simulink model "spherical_wrist"  (R2024b)
settings: Solver=ode23t  StartTime=0.0  StopTime=100  FixedStep=0.001  RelTol=1e-3
InitFcn:
  | % WRIST_mk2_1_DataFile
  | IC_021_G_207_MECH_DataFile
model workspace (MAT data in the model file):
  Damp : Simulink.Parameter (value not decoded)
  Dm : Simulink.Parameter (value not decoded)
  Jm : Simulink.Parameter (value not decoded)
  Km : Simulink.Parameter (value not decoded)
  Tc : Simulink.Parameter (value not decoded)
symbols that are objects in the model workspace (value not decoded): Damp, Dm, Tc
undefined symbols (not defined in the file or in its folder): smiData, X, Y, Z
libraries: sm_lib x370, nesl_utility x32, fl_lib x15, sdl_lib x9, simulink_extras x4, simulink x3, sharedtransform x2, slpidlib x1
(part 10 of 10)

== system spherical_wrist/NewWrist21/ROD 3/SPINA ROD 3 ==
  ReferenceFrame : sm_lib/Frames and Transforms/Reference Frame
  Solid : sm_lib/Body Elements/File Solid  ExtGeomFileName=ic_021_p_196_prt.step  UnitType=FromFile  ExtGeomFileUnits=m  StepReaderType=HEX  ExportConvexHullGeometry=off  InertiaType=Custom  BasedOnType=DensityFromFile  Density=1000  DensityUnits=kg/m^3  Mass=smiData.Solid(5).mass  MassUnits=kg  CenterOfMass=smiData.Solid(5).CoM  CenterOfMassUnits=mm  MomentsOfInertia=smiData.Solid(5).MoI  MomentsOfInertiaUnits=kg*mm^2  ProductsOfInertia=smiData.Solid(5).PoI  ProductsOfInertiaUnits=kg*mm^2  GraphicType=FromGeometry  MarkerShape=Sphere  MarkerSize=10  GraphicVisPropType=SimpleVisualProperties  GraphicDiffuseColor=smiData.Solid(5).color  GraphicOpacity=smiData.Solid(5).opacity  GraphicSpecularColor=[0.5 0.5 0.5 1.0]  GraphicAmbientColor=[0.15 0.15 0.15 1.0]  GraphicEmissiveColor=[0.0 0.0 0.0 1.0]  GraphicShininess=75  DoExposeReferenceFrame=on  SerializedFrames=<Frames/>
  Transform : sm_lib/Frames and Transforms/Rigid Transform  RotationMethod=ArbitraryAxis  FollAlignAxisA=+X  BaseAlignAxisA=+Y  FollAlignAxisB=+Y  BaseAlignAxisB=+Z  RotationStandardAxis=+Z  RotationAngle=smiData.RigidTransform(8).angle  RotationAngleUnits=rad  RotationArbitraryAxis=smiData.RigidTransform(8).axis  RotationSequenceAxes=FollowerAxes  RotationSequence=XYX  RotationSequenceAngles=[0 0 0]  RotationSequenceAnglesUnits=deg  RotationMatrix=[1 0 0;0 1 0;0 0 1]  Quaternion=[1 0 0 0]  TranslationMethod=Cartesian  TranslationCartesianOffset=smiData.RigidTransform(8).translation  TranslationCartesianOffsetUnits=mm  TranslationStandardAxis=+Z  TranslationStandardOffset=0  TranslationStandardOffsetUnits=m  TranslationROffset=0  TranslationROffsetUnits=m  TranslationThetaOffset=0  TranslationThetaOffsetUnits=deg  TranslationZOffset=0  TranslationZOffsetUnits=m
  F : PMIOPort  Side=Left
  connections:
  Solid/RConn1 -- ReferenceFrame/RConn1 -- Transform/LConn1
  Transform/RConn1 -- F/RConn1

== system spherical_wrist/NewWrist21/ROD 3/x618_4_RIGID ==
  ReferenceFrame : sm_lib/Frames and Transforms/Reference Frame
  Solid : sm_lib/Body Elements/File Solid  ExtGeomFileName=618-4_prt.step  UnitType=FromFile  ExtGeomFileUnits=m  StepReaderType=HEX  ExportConvexHullGeometry=off  InertiaType=Custom  BasedOnType=DensityFromFile  Density=1000  DensityUnits=kg/m^3  Mass=smiData.Solid(4).mass  MassUnits=kg  CenterOfMass=smiData.Solid(4).CoM  CenterOfMassUnits=mm  MomentsOfInertia=smiData.Solid(4).MoI  MomentsOfInertiaUnits=kg*mm^2  ProductsOfInertia=smiData.Solid(4).PoI  ProductsOfInertiaUnits=kg*mm^2  GraphicType=FromGeometry  MarkerShape=Sphere  MarkerSize=10  GraphicVisPropType=SimpleVisualProperties  GraphicDiffuseColor=smiData.Solid(4).color  GraphicOpacity=smiData.Solid(4).opacity  GraphicSpecularColor=[0.5 0.5 0.5 1.0]  GraphicAmbientColor=[0.15 0.15 0.15 1.0]  GraphicEmissiveColor=[0.0 0.0 0.0 1.0]  GraphicShininess=75  DoExposeReferenceFrame=on  SerializedFrames=<Frames/>
  F : PMIOPort  Side=Left
  connections:
  Solid/RConn1 -- ReferenceFrame/RConn1 -- F/RConn1

== system spherical_wrist/NewWrist21/ROD 3/x618_4_RIGID1 ==
  ReferenceFrame : sm_lib/Frames and Transforms/Reference Frame
  Solid : sm_lib/Body Elements/File Solid  ExtGeomFileName=618-4_prt.step  UnitType=FromFile  ExtGeomFileUnits=m  StepReaderType=HEX  ExportConvexHullGeometry=off  InertiaType=Custom  BasedOnType=DensityFromFile  Density=1000  DensityUnits=kg/m^3  Mass=smiData.Solid(4).mass  MassUnits=kg  CenterOfMass=smiData.Solid(4).CoM  CenterOfMassUnits=mm  MomentsOfInertia=smiData.Solid(4).MoI  MomentsOfInertiaUnits=kg*mm^2  ProductsOfInertia=smiData.Solid(4).PoI  ProductsOfInertiaUnits=kg*mm^2  GraphicType=FromGeometry  MarkerShape=Sphere  MarkerSize=10  GraphicVisPropType=SimpleVisualProperties  GraphicDiffuseColor=smiData.Solid(4).color  GraphicOpacity=smiData.Solid(4).opacity  GraphicSpecularColor=[0.5 0.5 0.5 1.0]  GraphicAmbientColor=[0.15 0.15 0.15 1.0]  GraphicEmissiveColor=[0.0 0.0 0.0 1.0]  GraphicShininess=75  DoExposeReferenceFrame=on  SerializedFrames=<Frames/>
  F : PMIOPort  Side=Left
  connections:
  Solid/RConn1 -- ReferenceFrame/RConn1 -- F/RConn1

== system spherical_wrist/NewWrist21/ROD 3/x618_4_RIGID2 ==
  ReferenceFrame : sm_lib/Frames and Transforms/Reference Frame
  Solid : sm_lib/Body Elements/File Solid  ExtGeomFileName=618-4_prt.step  UnitType=FromFile  ExtGeomFileUnits=m  StepReaderType=HEX  ExportConvexHullGeometry=off  InertiaType=Custom  BasedOnType=DensityFromFile  Density=1000  DensityUnits=kg/m^3  Mass=smiData.Solid(4).mass  MassUnits=kg  CenterOfMass=smiData.Solid(4).CoM  CenterOfMassUnits=mm  MomentsOfInertia=smiData.Solid(4).MoI  MomentsOfInertiaUnits=kg*mm^2  ProductsOfInertia=smiData.Solid(4).PoI  ProductsOfInertiaUnits=kg*mm^2  GraphicType=FromGeometry  MarkerShape=Sphere  MarkerSize=10  GraphicVisPropType=SimpleVisualProperties  GraphicDiffuseColor=smiData.Solid(4).color  GraphicOpacity=smiData.Solid(4).opacity  GraphicSpecularColor=[0.5 0.5 0.5 1.0]  GraphicAmbientColor=[0.15 0.15 0.15 1.0]  GraphicEmissiveColor=[0.0 0.0 0.0 1.0]  GraphicShininess=75  DoExposeReferenceFrame=on  SerializedFrames=<Frames/>
  Transform : sm_lib/Frames and Transforms/Rigid Transform  RotationMethod=ArbitraryAxis  FollAlignAxisA=+X  BaseAlignAxisA=+Y  FollAlignAxisB=+Y  BaseAlignAxisB=+Z  RotationStandardAxis=+Z  RotationAngle=smiData.RigidTransform(34).angle  RotationAngleUnits=rad  RotationArbitraryAxis=smiData.RigidTransform(34).axis  RotationSequenceAxes=FollowerAxes  RotationSequence=XYX  RotationSequenceAngles=[0 0 0]  RotationSequenceAnglesUnits=deg  RotationMatrix=[1 0 0;0 1 0;0 0 1]  Quaternion=[1 0 0 0]  TranslationMethod=Cartesian  TranslationCartesianOffset=smiData.RigidTransform(34).translation  TranslationCartesianOffsetUnits=mm  TranslationStandardAxis=+Z  TranslationStandardOffset=0  TranslationStandardOffsetUnits=m  TranslationROffset=0  TranslationROffsetUnits=m  TranslationThetaOffset=0  TranslationThetaOffsetUnits=deg  TranslationZOffset=0  TranslationZOffsetUnits=m
  Transform1 : sm_lib/Frames and Transforms/Rigid Transform  RotationMethod=ArbitraryAxis  FollAlignAxisA=+X  BaseAlignAxisA=+Y  FollAlignAxisB=+Y  BaseAlignAxisB=+Z  RotationStandardAxis=+Z  RotationAngle=smiData.RigidTransform(51).angle  RotationAngleUnits=rad  RotationArbitraryAxis=smiData.RigidTransform(51).axis  RotationSequenceAxes=FollowerAxes  RotationSequence=XYX  RotationSequenceAngles=[0 0 0]  RotationSequenceAnglesUnits=deg  RotationMatrix=[1 0 0;0 1 0;0 0 1]  Quaternion=[1 0 0 0]  TranslationMethod=Cartesian  TranslationCartesianOffset=smiData.RigidTransform(51).translation  TranslationCartesianOffsetUnits=mm  TranslationStandardAxis=+Z  TranslationStandardOffset=0  TranslationStandardOffsetUnits=m  TranslationROffset=0  TranslationROffsetUnits=m  TranslationThetaOffset=0  TranslationThetaOffsetUnits=deg  TranslationZOffset=0  TranslationZOffsetUnits=m
  F1 : PMIOPort  Side=Left
  F : PMIOPort  Port=2  Side=Left
  connections:
  Solid/RConn1 -- ReferenceFrame/RConn1 -- Transform/LConn1 -- Transform1/LConn1
  Transform/RConn1 -- F/RConn1
  Transform1/RConn1 -- F1/RConn1

== system spherical_wrist/NewWrist21/ROD 3/x618_4_RIGID3 ==
  ReferenceFrame : sm_lib/Frames and Transforms/Reference Frame
  Solid : sm_lib/Body Elements/File Solid  ExtGeomFileName=618-4_prt.step  UnitType=FromFile  ExtGeomFileUnits=m  StepReaderType=HEX  ExportConvexHullGeometry=off  InertiaType=Custom  BasedOnType=DensityFromFile  Density=1000  DensityUnits=kg/m^3  Mass=smiData.Solid(4).mass  MassUnits=kg  CenterOfMass=smiData.Solid(4).CoM  CenterOfMassUnits=mm  MomentsOfInertia=smiData.Solid(4).MoI  MomentsOfInertiaUnits=kg*mm^2  ProductsOfInertia=smiData.Solid(4).PoI  ProductsOfInertiaUnits=kg*mm^2  GraphicType=FromGeometry  MarkerShape=Sphere  MarkerSize=10  GraphicVisPropType=SimpleVisualProperties  GraphicDiffuseColor=smiData.Solid(4).color  GraphicOpacity=smiData.Solid(4).opacity  GraphicSpecularColor=[0.5 0.5 0.5 1.0]  GraphicAmbientColor=[0.15 0.15 0.15 1.0]  GraphicEmissiveColor=[0.0 0.0 0.0 1.0]  GraphicShininess=75  DoExposeReferenceFrame=on  SerializedFrames=<Frames/>
  Transform : sm_lib/Frames and Transforms/Rigid Transform  RotationMethod=ArbitraryAxis  FollAlignAxisA=+X  BaseAlignAxisA=+Y  FollAlignAxisB=+Y  BaseAlignAxisB=+Z  RotationStandardAxis=+Z  RotationAngle=smiData.RigidTransform(46).angle  RotationAngleUnits=rad  RotationArbitraryAxis=smiData.RigidTransform(46).axis  RotationSequenceAxes=FollowerAxes  RotationSequence=XYX  RotationSequenceAngles=[0 0 0]  RotationSequenceAnglesUnits=deg  RotationMatrix=[1 0 0;0 1 0;0 0 1]  Quaternion=[1 0 0 0]  TranslationMethod=Cartesian  TranslationCartesianOffset=smiData.RigidTransform(46).translation  TranslationCartesianOffsetUnits=mm  TranslationStandardAxis=+Z  TranslationStandardOffset=0  TranslationStandardOffsetUnits=m  TranslationROffset=0  TranslationROffsetUnits=m  TranslationThetaOffset=0  TranslationThetaOffsetUnits=deg  TranslationZOffset=0  TranslationZOffsetUnits=m
  Transform1 : sm_lib/Frames and Transforms/Rigid Transform  RotationMethod=ArbitraryAxis  FollAlignAxisA=+X  BaseAlignAxisA=+Y  FollAlignAxisB=+Y  BaseAlignAxisB=+Z  RotationStandardAxis=+Z  RotationAngle=smiData.RigidTransform(57).angle  RotationAngleUnits=rad  RotationArbitraryAxis=smiData.RigidTransform(57).axis  RotationSequenceAxes=FollowerAxes  RotationSequence=XYX  RotationSequenceAngles=[0 0 0]  RotationSequenceAnglesUnits=deg  RotationMatrix=[1 0 0;0 1 0;0 0 1]  Quaternion=[1 0 0 0]  TranslationMethod=Cartesian  TranslationCartesianOffset=smiData.RigidTransform(57).translation  TranslationCartesianOffsetUnits=mm  TranslationStandardAxis=+Z  TranslationStandardOffset=0  TranslationStandardOffsetUnits=m  TranslationROffset=0  TranslationROffsetUnits=m  TranslationThetaOffset=0  TranslationThetaOffsetUnits=deg  TranslationZOffset=0  TranslationZOffsetUnits=m
  F1 : PMIOPort  Side=Left
  F : PMIOPort  Port=2  Side=Left
  connections:
  Solid/RConn1 -- ReferenceFrame/RConn1 -- Transform/LConn1 -- Transform1/LConn1
  Transform/RConn1 -- F/RConn1
  Transform1/RConn1 -- F1/RConn1

== system spherical_wrist/Position_Controller/wrapTo180Simulink/singleWrapTo180_1 ==
  angle : Inport
  Add6 : Sum  Inputs=-+
  Add7 : Sum
  Constant : Constant  Value=360
  Constant4 : Constant  Value=180
  Constant5 : Constant  Value=360
  Constant6 : Constant  Value=-180
  Relational Operator : RelationalOperator  Operator=>  OutDataTypeStr=boolean  RndMeth=Simplest  InputSameDT=off
  Relational Operator1 : RelationalOperator  Operator=<  OutDataTypeStr=boolean  RndMeth=Simplest  InputSameDT=off
  Switch4 : Switch  Criteria=u2 > Threshold  SaturateOnIntegerOverflow=off  InputSameDT=off
  Switch5 : Switch  Criteria=u2 > Threshold  SaturateOnIntegerOverflow=off  InputSameDT=off
  wrappedAngle : Outport
  wires:
  Relational Operator/1 -> Switch4/2
  Constant5/1 -> Add6/1
  Switch5/1 -> wrappedAngle/1
  Add7/1 -> Switch5/1
  Constant4/1 -> Relational Operator/2
  Switch4/1 -> Switch5/3
  Constant/1 -> Add7/2
  Add6/1 -> Switch4/1
  angle/1 -> Switch4/3, Relational Operator/1, Add6/2, Add7/1, Relational Operator1/1
  Constant6/1 -> Relational Operator1/2
  Relational Operator1/1 -> Switch5/2

== system spherical_wrist/Position_Controller/wrapTo180Simulink/singleWrapTo180_2 ==
  angle : Inport
  Add6 : Sum  Inputs=-+
  Add7 : Sum
  Constant : Constant  Value=360
  Constant4 : Constant  Value=180
  Constant5 : Constant  Value=360
  Constant6 : Constant  Value=-180
  Relational Operator : RelationalOperator  Operator=>  OutDataTypeStr=boolean  RndMeth=Simplest  InputSameDT=off
  Relational Operator1 : RelationalOperator  Operator=<  OutDataTypeStr=boolean  RndMeth=Simplest  InputSameDT=off
  Switch4 : Switch  Criteria=u2 > Threshold  SaturateOnIntegerOverflow=off  InputSameDT=off
  Switch5 : Switch  Criteria=u2 > Threshold  SaturateOnIntegerOverflow=off  InputSameDT=off
  wrappedAngle : Outport
  wires:
  Relational Operator/1 -> Switch4/2
  Constant5/1 -> Add6/1
  Switch5/1 -> wrappedAngle/1
  Add7/1 -> Switch5/1
  Constant4/1 -> Relational Operator/2
  Switch4/1 -> Switch5/3
  Constant/1 -> Add7/2
  Add6/1 -> Switch4/1
  angle/1 -> Switch4/3, Relational Operator/1, Add6/2, Add7/1, Relational Operator1/1
  Constant6/1 -> Relational Operator1/2
  Relational Operator1/1 -> Switch5/2

== system spherical_wrist/Position_Controller/wrapTo180Simulink/singleWrapTo180_3 ==
  angle : Inport
  Add6 : Sum  Inputs=-+
  Add7 : Sum
  Constant : Constant  Value=360
  Constant4 : Constant  Value=180
  Constant5 : Constant  Value=360
  Constant6 : Constant  Value=-180
  Relational Operator : RelationalOperator  Operator=>  OutDataTypeStr=boolean  RndMeth=Simplest  InputSameDT=off
  Relational Operator1 : RelationalOperator  Operator=<  OutDataTypeStr=boolean  RndMeth=Simplest  InputSameDT=off
  Switch4 : Switch  Criteria=u2 > Threshold  SaturateOnIntegerOverflow=off  InputSameDT=off
  Switch5 : Switch  Criteria=u2 > Threshold  SaturateOnIntegerOverflow=off  InputSameDT=off
  wrappedAngle : Outport
  wires:
  Relational Operator/1 -> Switch4/2
  Constant5/1 -> Add6/1
  Switch5/1 -> wrappedAngle/1
  Add7/1 -> Switch5/1
  Constant4/1 -> Relational Operator/2
  Switch4/1 -> Switch5/3
  Constant/1 -> Add7/2
  Add6/1 -> Switch4/1
  angle/1 -> Switch4/3, Relational Operator/1, Add6/2, Add7/1, Relational Operator1/1
  Constant6/1 -> Relational Operator1/2
  Relational Operator1/1 -> Switch5/2

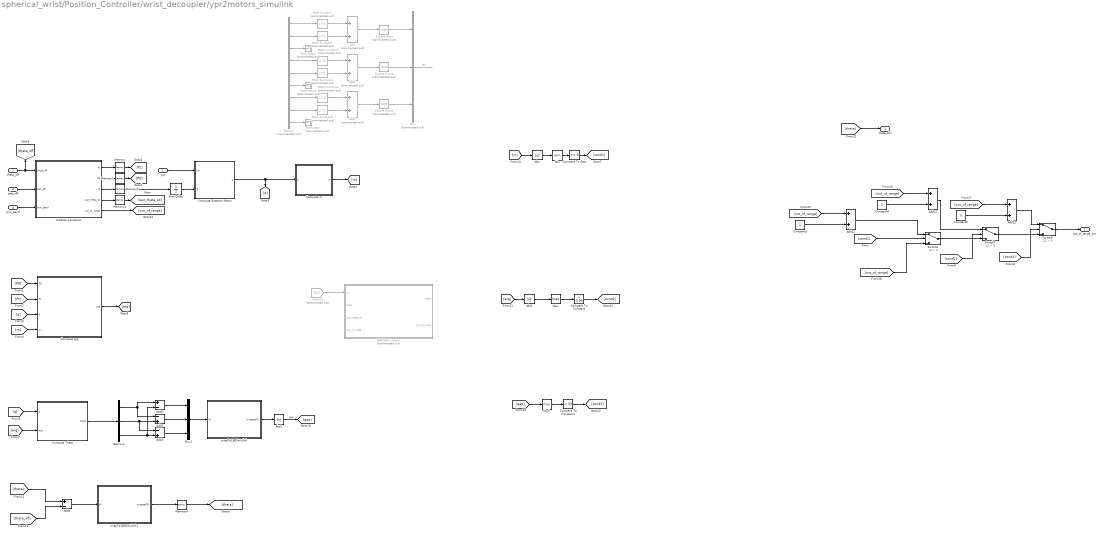
== system spherical_wrist/Position_Controller/wrist_decoupler/ypr2motors_simulink ==
  ypr : Inport
  theta_off : Inport  Port=2
  plat_off : Inport  Port=3
  arm_bend : Inport  Port=4
  Abs : Abs  SaturateOnIntegerOverflow=off
  Abs1 : Abs  SaturateOnIntegerOverflow=off
  Abs2 : Abs  SaturateOnIntegerOverflow=off
  Add : Sum  Commented=on
  Add1 : Sum  Commented=on
  Add11 : Sum
  Add12 : Sum
  Add13 : Sum
  Add2 : Sum  Commented=on
  Add3 : Sum  Inputs=-+
  Add4 : Sum  Inputs=-+
  Add5 : Sum  Inputs=+-
  Add6 : Sum  Inputs=+-
  Compare To Constant : simulink/Logic and Bit Operations/Compare To Constant  relop=>  const=0.99  OutDataTypeStr=boolean
  Compare To Constant1 : simulink/Logic and Bit Operations/Compare To Constant  relop=<  const=33  OutDataTypeStr=boolean
  Compare To Zero : simulink/Logic and Bit Operations/Compare To Zero  relop===  OutDataTypeStr=boolean
  Compute Rotation Matrix : MATLAB Function  TreatAsAtomicUnit=on
      settings: MinAlgLoopOccurrences=on
  Compute Theta : MATLAB Function  TreatAsAtomicUnit=on
  Compute arg : MATLAB Function  TreatAsAtomicUnit=on
      settings: MinAlgLoopOccurrences=on
  Compute m : MATLAB Function  TreatAsAtomicUnit=on
  Constant3 : Constant
  Constant4 : Constant  Value=2
  Constant5 : Constant  Value=3
  Demux : Demux  Commented=on  Outputs=9
  Demux1 : Demux  Outputs=3
  From24 : From  Commented=on  GotoTag=m
  Initialize Constants : MATLAB Function  TreatAsAtomicUnit=on
      settings: MinAlgLoopOccurrences=on
  MATLAB Function : MATLAB Function  Commented=on  TreatAsAtomicUnit=on
  Math Function{,1..5} (6 alike) : Math  Commented=on  Operator=square
  Max : MinMax  Function=max
  Memory{,1..4} (5 alike) : Memory  InheritSampleTime=on
  Min : MinMax
  Min1 : MinMax
  Mux : Mux  Commented=on  Inputs=3
  Mux1 : Mux  Inputs=3
  Square Root : Sqrt  Commented=on
  Square Root1 : Sqrt  Commented=on
  Square Root2 : Sqrt  Commented=on
  Switch6 : Switch  Criteria=u2 > Threshold  SaturateOnIntegerOverflow=off  InputSameDT=off
  Switch7 : Switch  Criteria=u2 > Threshold  SaturateOnIntegerOverflow=off  InputSameDT=off
  Switch8 : Switch  Criteria=u2 > Threshold  SaturateOnIntegerOverflow=off  InputSameDT=off
  Terminator : Terminator  Commented=on
  Terminator1 : Terminator  Commented=on
  Terminator2 : Terminator  Commented=on
  Unit Delay : UnitDelay  SampleTime=-1  HasFrameUpgradeWarning=on
  wrapTo180Simulink : Subsystem
  wrapTo180Simulink1 : Subsystem
  theta_sim : Outport
  out_of_range_sim : Outport  Port=2
  wires:
  theta_off/1 -> Initialize Constants/1(theta_off), [theta_off]
  plat_off/1 -> Initialize Constants/2(plat_off)
  arm_bend/1 -> Initialize Constants/3(arm_bend)
  Initialize Constants/1(Pz) -> Memory/1
  Initialize Constants/2(PQ) -> Memory1/1
  Initialize Constants/3(Q) -> Memory2/1
  ypr/1 -> Compute Rotation Matrix/1(ypr)
  Memory2/1 -> Unit Delay/1
  Memory1/1 -> [PQ]
  Memory/1 -> [Pz]
  [Pz] -> Compute arg/2(Pz)
  Compute Rotation Matrix/1(q) -> Compute m/1(q), [q]
  [q] -> Compute arg/3(q)
  [m] -> Compute arg/4(m)
  Compute arg/1(arg) -> [arg]
  [q] -> Compute Theta/1(q)
  [arg] -> Compute Theta/2(arg)
  Compute Theta/1(theta) -> Demux1/1
  Demux1/2 -> Add4/1, Add3/2
  Demux1/1 -> Add3/1, Add5/1
  Demux1/3 -> Add5/2, Add4/2
  Add5/1 -> Mux1/1
  Add3/1 -> Mux1/2
  Add4/1 -> Mux1/3
  Mux1/1 -> wrapTo180Simulink/1(th)
  [theta] -> Add6/1
  [theta_off] -> Add6/2
  Add6/1 -> wrapTo180Simulink1/1(th)
  wrapTo180Simulink1/1(wrappedTh) -> Memory4/1
  Memory4/1 -> [theta]
  Initialize Constants/4(last_theta_ok) -> Memory3/1
  Memory3/1 -> [last_theta_ok]
  [theta] -> theta_sim/1
  Initialize Constants/5(out_of_range) -> [out_of_range]
  Min/1 -> Compare To Zero/1
  Compare To Zero/1 -> [cond1]
  Abs/1 -> Min/1
  [m] -> Abs/1
  Abs1/1 -> Max/1
  Max/1 -> Compare To Constant/1
  Compare To Constant/1 -> [cond2]
  [arg] -> Abs1/1
  Min1/1 -> Compare To Constant1/1
  Compare To Constant1/1 -> [cond3]
  wrapTo180Simulink/1(wrappedTh) -> Abs2/1
  Abs2/1 -> [gap]  "gap"
  [gap] -> Min1/1
  From24/1 -> MATLAB Function/1(m)
  Constant3/1 -> Add11/2
  [out_of_range] -> Add11/1
  Add11/1 -> Switch6/1
  Switch6/1 -> Switch7/3
  Switch7/1 -> Switch8/3
  [out_of_range] -> Add12/1
  Add12/1 -> Switch7/1
  Constant4/1 -> Add12/2
  [out_of_range] -> Add13/1
  Add13/1 -> Switch8/1
  Constant5/1 -> Add13/2
  Switch8/1 -> out_of_range_sim/1
  [out_of_range] -> Switch6/3
  [cond1] -> Switch6/2
  [cond2] -> Switch7/2
  [cond3] -> Switch8/2
  Add/1 -> Square Root/1
  Square Root1/1 -> Mux/2
  Demux/3 -> Terminator2/1
  Demux/9 -> Terminator/1
  Square Root/1 -> Mux/1
  Square Root2/1 -> Mux/3
  Math Function/1 -> Add/1
  Math Function1/1 -> Add/2
  Demux/6 -> Terminator1/1
  Math Function2/1 -> Add1/1
  Mux/1 -> ?  "m"
  Demux/7 -> Math Function4/1
  Demux/4 -> Math Function2/1
  Demux/8 -> Math Function5/1
  Demux/1 -> Math Function/1
  Demux/5 -> Math Function3/1
  Math Function4/1 -> Add2/1
  Math Function3/1 -> Add1/2
  ? -> Demux/1
  Add1/1 -> Square Root1/1
  Add2/1 -> Square Root2/1
  Demux/2 -> Math Function1/1
  Math Function5/1 -> Add2/2
  Compute m/1(m) -> [m]
  Unit Delay/1 -> Compute Rotation Matrix/2(Q)
  [PQ] -> Compute arg/1(PQ)

== system spherical_wrist/Position_Controller/wrist_decoupler/ypr2motors_simulink/wrapTo180Simulink ==
  th : Inport
  Demux : Demux  Outputs=3
  Mux : Mux  Inputs=3
  singleWrapTo180_1 : Subsystem
  singleWrapTo180_2 : Subsystem
  singleWrapTo180_3 : Subsystem
  wrappedTh : Outport
  wires:
  singleWrapTo180_1/1(wrappedAngle) -> Mux/1
  singleWrapTo180_3/1(wrappedAngle) -> Mux/3
  singleWrapTo180_2/1(wrappedAngle) -> Mux/2
  Demux/3 -> singleWrapTo180_3/1(angle)
  th/1 -> Demux/1
  Demux/1 -> singleWrapTo180_1/1(angle)
  Demux/2 -> singleWrapTo180_2/1(angle)
  Mux/1 -> wrappedTh/1

== system spherical_wrist/Position_Controller/wrist_decoupler/ypr2motors_simulink/wrapTo180Simulink1 ==
  th : Inport
  Demux : Demux  Outputs=3
  Mux : Mux  Inputs=3
  singleWrapTo180_1 : Subsystem
  singleWrapTo180_2 : Subsystem
  singleWrapTo180_3 : Subsystem
  wrappedTh : Outport
  wires:
  singleWrapTo180_1/1(wrappedAngle) -> Mux/1
  singleWrapTo180_3/1(wrappedAngle) -> Mux/3
  singleWrapTo180_2/1(wrappedAngle) -> Mux/2
  Demux/3 -> singleWrapTo180_3/1(angle)
  th/1 -> Demux/1
  Demux/1 -> singleWrapTo180_1/1(angle)
  Demux/2 -> singleWrapTo180_2/1(angle)
  Mux/1 -> wrappedTh/1

== system spherical_wrist/Position_Controller/wrist_decoupler/ypr2motors_simulink/wrapTo180Simulink/singleWrapTo180_1 ==
  angle : Inport
  Add6 : Sum  Inputs=-+
  Add7 : Sum
  Constant : Constant  Value=360
  Constant4 : Constant  Value=180
  Constant5 : Constant  Value=360
  Constant6 : Constant  Value=-180
  Relational Operator : RelationalOperator  Operator=>  OutDataTypeStr=boolean  RndMeth=Simplest  InputSameDT=off
  Relational Operator1 : RelationalOperator  Operator=<  OutDataTypeStr=boolean  RndMeth=Simplest  InputSameDT=off
  Switch4 : Switch  Criteria=u2 > Threshold  SaturateOnIntegerOverflow=off  InputSameDT=off
  Switch5 : Switch  Criteria=u2 > Threshold  SaturateOnIntegerOverflow=off  InputSameDT=off
  wrappedAngle : Outport
  wires:
  Relational Operator/1 -> Switch4/2
  Constant5/1 -> Add6/1
  Switch5/1 -> wrappedAngle/1
  Add7/1 -> Switch5/1
  Constant4/1 -> Relational Operator/2
  Switch4/1 -> Switch5/3
  Constant/1 -> Add7/2
  Add6/1 -> Switch4/1
  angle/1 -> Switch4/3, Relational Operator/1, Add6/2, Add7/1, Relational Operator1/1
  Constant6/1 -> Relational Operator1/2
  Relational Operator1/1 -> Switch5/2

== system spherical_wrist/Position_Controller/wrist_decoupler/ypr2motors_simulink/wrapTo180Simulink/singleWrapTo180_2 ==
  angle : Inport
  Add6 : Sum  Inputs=-+
  Add7 : Sum
  Constant : Constant  Value=360
  Constant4 : Constant  Value=180
  Constant5 : Constant  Value=360
  Constant6 : Constant  Value=-180
  Relational Operator : RelationalOperator  Operator=>  OutDataTypeStr=boolean  RndMeth=Simplest  InputSameDT=off
  Relational Operator1 : RelationalOperator  Operator=<  OutDataTypeStr=boolean  RndMeth=Simplest  InputSameDT=off
  Switch4 : Switch  Criteria=u2 > Threshold  SaturateOnIntegerOverflow=off  InputSameDT=off
  Switch5 : Switch  Criteria=u2 > Threshold  SaturateOnIntegerOverflow=off  InputSameDT=off
  wrappedAngle : Outport
  wires:
  Relational Operator/1 -> Switch4/2
  Constant5/1 -> Add6/1
  Switch5/1 -> wrappedAngle/1
  Add7/1 -> Switch5/1
  Constant4/1 -> Relational Operator/2
  Switch4/1 -> Switch5/3
  Constant/1 -> Add7/2
  Add6/1 -> Switch4/1
  angle/1 -> Switch4/3, Relational Operator/1, Add6/2, Add7/1, Relational Operator1/1
  Constant6/1 -> Relational Operator1/2
  Relational Operator1/1 -> Switch5/2

== system spherical_wrist/Position_Controller/wrist_decoupler/ypr2motors_simulink/wrapTo180Simulink/singleWrapTo180_3 ==
  angle : Inport
  Add6 : Sum  Inputs=-+
  Add7 : Sum
  Constant : Constant  Value=360
  Constant4 : Constant  Value=180
  Constant5 : Constant  Value=360
  Constant6 : Constant  Value=-180
  Relational Operator : RelationalOperator  Operator=>  OutDataTypeStr=boolean  RndMeth=Simplest  InputSameDT=off
  Relational Operator1 : RelationalOperator  Operator=<  OutDataTypeStr=boolean  RndMeth=Simplest  InputSameDT=off
  Switch4 : Switch  Criteria=u2 > Threshold  SaturateOnIntegerOverflow=off  InputSameDT=off
  Switch5 : Switch  Criteria=u2 > Threshold  SaturateOnIntegerOverflow=off  InputSameDT=off
  wrappedAngle : Outport
  wires:
  Relational Operator/1 -> Switch4/2
  Constant5/1 -> Add6/1
  Switch5/1 -> wrappedAngle/1
  Add7/1 -> Switch5/1
  Constant4/1 -> Relational Operator/2
  Switch4/1 -> Switch5/3
  Constant/1 -> Add7/2
  Add6/1 -> Switch4/1
  angle/1 -> Switch4/3, Relational Operator/1, Add6/2, Add7/1, Relational Operator1/1
  Constant6/1 -> Relational Operator1/2
  Relational Operator1/1 -> Switch5/2

== system spherical_wrist/Position_Controller/wrist_decoupler/ypr2motors_simulink/wrapTo180Simulink1/singleWrapTo180_1 ==
  angle : Inport
  Add6 : Sum  Inputs=-+
  Add7 : Sum
  Constant : Constant  Value=360
  Constant4 : Constant  Value=180
  Constant5 : Constant  Value=360
  Constant6 : Constant  Value=-180
  Relational Operator : RelationalOperator  Operator=>  OutDataTypeStr=boolean  RndMeth=Simplest  InputSameDT=off
  Relational Operator1 : RelationalOperator  Operator=<  OutDataTypeStr=boolean  RndMeth=Simplest  InputSameDT=off
  Switch4 : Switch  Criteria=u2 > Threshold  SaturateOnIntegerOverflow=off  InputSameDT=off
  Switch5 : Switch  Criteria=u2 > Threshold  SaturateOnIntegerOverflow=off  InputSameDT=off
  wrappedAngle : Outport
  wires:
  Relational Operator/1 -> Switch4/2
  Constant5/1 -> Add6/1
  Switch5/1 -> wrappedAngle/1
  Add7/1 -> Switch5/1
  Constant4/1 -> Relational Operator/2
  Switch4/1 -> Switch5/3
  Constant/1 -> Add7/2
  Add6/1 -> Switch4/1
  angle/1 -> Switch4/3, Relational Operator/1, Add6/2, Add7/1, Relational Operator1/1
  Constant6/1 -> Relational Operator1/2
  Relational Operator1/1 -> Switch5/2

== system spherical_wrist/Position_Controller/wrist_decoupler/ypr2motors_simulink/wrapTo180Simulink1/singleWrapTo180_2 ==
  angle : Inport
  Add6 : Sum  Inputs=-+
  Add7 : Sum
  Constant : Constant  Value=360
  Constant4 : Constant  Value=180
  Constant5 : Constant  Value=360
  Constant6 : Constant  Value=-180
  Relational Operator : RelationalOperator  Operator=>  OutDataTypeStr=boolean  RndMeth=Simplest  InputSameDT=off
  Relational Operator1 : RelationalOperator  Operator=<  OutDataTypeStr=boolean  RndMeth=Simplest  InputSameDT=off
  Switch4 : Switch  Criteria=u2 > Threshold  SaturateOnIntegerOverflow=off  InputSameDT=off
  Switch5 : Switch  Criteria=u2 > Threshold  SaturateOnIntegerOverflow=off  InputSameDT=off
  wrappedAngle : Outport
  wires:
  Relational Operator/1 -> Switch4/2
  Constant5/1 -> Add6/1
  Switch5/1 -> wrappedAngle/1
  Add7/1 -> Switch5/1
  Constant4/1 -> Relational Operator/2
  Switch4/1 -> Switch5/3
  Constant/1 -> Add7/2
  Add6/1 -> Switch4/1
  angle/1 -> Switch4/3, Relational Operator/1, Add6/2, Add7/1, Relational Operator1/1
  Constant6/1 -> Relational Operator1/2
  Relational Operator1/1 -> Switch5/2

== system spherical_wrist/Position_Controller/wrist_decoupler/ypr2motors_simulink/wrapTo180Simulink1/singleWrapTo180_3 ==
  angle : Inport
  Add6 : Sum  Inputs=-+
  Add7 : Sum
  Constant : Constant  Value=360
  Constant4 : Constant  Value=180
  Constant5 : Constant  Value=360
  Constant6 : Constant  Value=-180
  Relational Operator : RelationalOperator  Operator=>  OutDataTypeStr=boolean  RndMeth=Simplest  InputSameDT=off
  Relational Operator1 : RelationalOperator  Operator=<  OutDataTypeStr=boolean  RndMeth=Simplest  InputSameDT=off
  Switch4 : Switch  Criteria=u2 > Threshold  SaturateOnIntegerOverflow=off  InputSameDT=off
  Switch5 : Switch  Criteria=u2 > Threshold  SaturateOnIntegerOverflow=off  InputSameDT=off
  wrappedAngle : Outport
  wires:
  Relational Operator/1 -> Switch4/2
  Constant5/1 -> Add6/1
  Switch5/1 -> wrappedAngle/1
  Add7/1 -> Switch5/1
  Constant4/1 -> Relational Operator/2
  Switch4/1 -> Switch5/3
  Constant/1 -> Add7/2
  Add6/1 -> Switch4/1
  angle/1 -> Switch4/3, Relational Operator/1, Add6/2, Add7/1, Relational Operator1/1
  Constant6/1 -> Relational Operator1/2
  Relational Operator1/1 -> Switch5/2

== matlab function spherical_wrist/Position_Controller/wrist_decoupler/ypr2motors_simulink/Compute m ==
  data: q input; m output
function m = compute_m(q)
m = [sqrt(q(1,1)^2+q(1,2)^2) sqrt(q(2,1)^2+q(2,2)^2) sqrt(q(3,1)^2+q(3,2)^2)];
end

== matlab function spherical_wrist/Position_Controller/wrapTo180 ==
  data: u input; y output
function y = wrap(u)

y = u;

for i=1:3
    while y(i) > 180.0
        y(i) = y(i) - 360.0;
    end

    while y(i) < -180.0
        y(i) = y(i) + 360.0;
    end
end

== matlab function spherical_wrist/Position_Controller/wrist_decoupler/ypr2motors ==
  data: ypr input; theta output; out_of_range output; theta_off input; plat_off input; arm_bend input
function [theta,out_of_range] = ypr2motors(ypr, theta_off, plat_off, arm_bend)

persistent Pz;
persistent PQ;
persistent Q;
persistent last_theta_ok;

if isempty(Pz)
    Pz = -tand(arm_bend)*[1; 1; 1];
    P = [cosd(theta_off) sind(theta_off) Pz];
    Q = [cosd(plat_off) sind(plat_off) [0; 0; 0]];
    PQ = [P(1,:)*Q(1,:)' P(2,:)*Q(2,:)' P(3,:)*Q(3,:)'];
    last_theta_ok = [0;0;0];
end

q = Q*eul2rotm(deg2rad(ypr'))';

m = [sqrt(q(1,1)^2+q(1,2)^2) sqrt(q(2,1)^2+q(2,2)^2) sqrt(q(3,1)^2+q(3,2)^2)];

if min(abs(m)) == 0
    % out of mechanical motion range
    theta = last_theta_ok;
    out_of_range = 1;
    return;
end

arg = [(PQ(1)-Pz(1)*q(1,3))/m(1); (PQ(2)-Pz(2)*q(2,3))/m(2); (PQ(3)-Pz(3)*q(3,3))/m(3)];

if max(abs(arg)) > 0.99
    % out of mechanical motion range
    theta = last_theta_ok;
    out_of_range = 2;
    return;
end

theta = atan2d(q(:,2),q(:,1))+[90; 90; 90;]-asind(arg);

gap = abs(Wrap180([(theta(2)-theta(1)) (theta(3)-theta(2)) (theta(1)-theta(3))]));

if min(gap) < 33.0
    % out of mechanical motion range
    theta = last_theta_ok;
    out_of_range = 3;
    return;
end

theta = Wrap180(theta-theta_off);

last_theta_ok = theta;
        
out_of_range = 0;

end

%%%%%%%%%%%%%%%%%%%%%%%

function y = Wrap180(x)

    y = x;

    for i=1:3
        while y(i) > 180.0
            y(i) = y(i) - 360.0;
        end
 
        while y(i) < -180.0
            y(i) = y(i) + 360.0;
        end
    end
end

== matlab function spherical_wrist/Position_Controller/wrist_decoupler/ypr2motors_simulink/Initialize Constants ==
  data: theta_off input; Pz output; plat_off input; arm_bend input; PQ output; Q output; last_theta_ok output; out_of_range output
function [Pz, PQ, Q, last_theta_ok, out_of_range] = initialize_constants(theta_off, plat_off, arm_bend)
Pz = -tand(arm_bend)*[1; 1; 1];
P = [cosd(theta_off) sind(theta_off) Pz];
Q = [cosd(plat_off) sind(plat_off) [0; 0; 0]];
PQ = [P(1,:)*Q(1,:)' P(2,:)*Q(2,:)' P(3,:)*Q(3,:)'];
last_theta_ok = [0;0;0];
out_of_range = 0;
end

== matlab function spherical_wrist/Position_Controller/wrist_decoupler/motors2ypr ==
  settings: sampleTime=0.1
  data: theta_diff input; theta_off input; attitude output; singularity output; cycles output; plat_off input; arm_bend input
function [attitude,singularity,cycles] = motors2ypr(theta_diff, theta_off, plat_off, arm_bend)

persistent Q;
persistent PQ;
persistent Pz;
persistent T;
persistent attitude_ok;

theta_diff = Wrap180(theta_diff);

if isempty(Q)
    Pz = -tand(arm_bend)*[1; 1; 1];
    P = [cosd(theta_off) sind(theta_off) Pz];
    Q = [cosd(plat_off) sind(plat_off) [0; 0; 0]];
    PQ = [P(1,:)*Q(1,:)' P(2,:)*Q(2,:)' P(3,:)*Q(3,:)'];

    hyaw = 0.1666*(theta_diff(1)+theta_diff(2)+theta_diff(3));
    T = quaternion(cosd(hyaw),0,0,sind(0.5*hyaw));
    attitude_ok = compact(T);
end

%%%%%%%%%%%%%%%%%%%%%%%%%%%%%%%%%%%%%%%%%%%%%%%%%%%%

%%%%%%%%%%%%%%%%%%%%%%%%%%%%%%%%%%%%%%%%%%%%%%%%%%%%

%hyaw = 0.1666*(theta_diff(1)+theta_diff(2)+theta_diff(3));
%T = quaternion(cosd(hyaw),0,0,sind(0.5*hyaw));
%T = quaternion(1,0,0,0);

Told = T;

singularity = 0;

step = 0.01;

first_try = true;

for cycles=1:40
    
    q = rotatepoint(T,Q);
    
    %%%%%%%%%%%%%%%%%%%%%%%%%%%%%%%%%%%%%%%%%%%%%%%%%%%%%%%%%%%%%%%%%%%%%%%
    
    m = [sqrt(q(1,1)^2+q(1,2)^2) sqrt(q(2,1)^2+q(2,2)^2) sqrt(q(3,1)^2+q(3,2)^2)];

    if min(abs(m)) == 0
        % out of mechanical motion range
        if step > 0.001
            step = 0.5*step;
            T = Told;
            continue;
        elseif first_try
            first_try = false;
            step = 0.01;
            hyaw = 0.1666*(theta_diff(1)+theta_diff(2)+theta_diff(3));
            T = quaternion(cosd(hyaw),0,0,sind(0.5*hyaw));
            continue;
        end
        
        break;
    end
    
    arg = [(PQ(1)-Pz(1)*q(1,3))/m(1); (PQ(2)-Pz(2)*q(2,3))/m(2); (PQ(3)-Pz(3)*q(3,3))/m(3)];
    
    if max(abs(arg)) > 1.0
        % out of mechanical motion range
        if step > 0.001
            step = 0.5*step;
            T = Told;
            continue;
        elseif first_try
            first_try = false;
            step = 0.01;
            hyaw = 0.1666*(theta_diff(1)+theta_diff(2)+theta_diff(3));
            T = quaternion(cosd(hyaw),0,0,sind(0.5*hyaw));
            continue;
        end

        break;
    end
    
    theta = atan2d(q(:,2),q(:,1))+[90; 90; 90;]-asind(arg);
    
    %%%%%%%%%%%%%%%%%%%%%%%%%%%%%%%%%%%%%%%%%%%%%%%%%%%%%%%%%%%%%%%%%%%%%%%
    
    theta_err = Wrap180(theta_diff+theta_off-theta);
       
    if max(abs(theta_err)) < 0.1
        T = normalize(T);
        attitude = compact(T);
        attitude_ok = attitude;
        return;
    end
        
    p = [cosd(theta) sind(theta) Pz];
        
    q1xp1 = cross(q(1,:),p(1,:));
    q2xp2 = cross(q(2,:),p(2,:));
    q3xp3 = cross(q(3,:),p(3,:));
        
    if min(abs([q1xp1(3) q2xp2(3) q3xp3(3)])) == 0.0
        % ill jacobian
        if step > 0.001
            step = 0.5*step;
            T = Told;
            continue;
        elseif first_try
            first_try = false;
            step = 0.01;
            hyaw = 0.1666*(theta_diff(1)+theta_diff(2)+theta_diff(3));
            T = quaternion(cosd(hyaw),0,0,sind(0.5*hyaw));
            continue;
        end

        break;
    end
        
    if det([q1xp1/q1xp1(3); q2xp2/q2xp2(3); q3xp3/q3xp3(3)]) == 0.0
        % ill jacobian
        if step > 0.001
            step = 0.5*step;
            T = Told;
            continue;
        elseif first_try
            first_try = false;
            step = 0.01;
            hyaw = 0.1666*(theta_diff(1)+theta_diff(2)+theta_diff(3));
            T = quaternion(cosd(hyaw),0,0,sind(0.5*hyaw));
            continue;
        end

        break;
    end
        
    Told = T;
    T = quaternion(([q1xp1/q1xp1(3); q2xp2/q2xp2(3); q3xp3/q3xp3(3)]\(step*theta_err))','rotvec')*T;
end

T = quaternion(1,0,0,0);
attitude = attitude_ok;
singularity = 1;

end

%%%%%%%%%%%%%%%%%%%%%%%

function y = Wrap180(x)

    y = x;

    for i=1:3
        while y(i) >= 180.0
            y(i) = y(i) - 360.0;
        end
 
        while y(i) < -180.0
            y(i) = y(i) + 360.0;
        end
    end
end

== matlab function spherical_wrist/Position_Controller/wrist_decoupler/ypr2motors_simulink/Compute Rotation Matrix ==
  data: ypr input; q output; Q input
function q = compute_rotation(ypr, Q)
q = Q * eul2rotm(deg2rad(ypr'))';
end

== matlab function spherical_wrist/Position_Controller/wrist_decoupler/ypr2motors_simulink/Compute arg ==
  data: PQ input; arg output; Pz input; q input; m input
function arg = compute_arg(PQ, Pz, q, m)
arg = [(PQ(1)-Pz(1)*q(1,3))/m(1); (PQ(2)-Pz(2)*q(2,3))/m(2); (PQ(3)-Pz(3)*q(3,3))/m(3)];
end

== matlab function spherical_wrist/Position_Controller/wrist_decoupler/ypr2motors_simulink/Compute Theta ==
  data: q input; theta output; arg input
function theta = compute_theta(q, arg)
theta = atan2d(q(:,2), q(:,1)) + [90; 90; 90] - asind(arg);
end

== matlab function spherical_wrist/Position_Controller/wrist_decoupler/ypr2motors_simulink/MATLAB Function ==
  data: m input; theta output; theta input; last_theta_ok input; out_of_range input; out_of_range output
function [theta, out_of_range]= fcn(m, theta, last_theta_ok, out_of_range)
% out of mechanical motion range
theta = last_theta_ok;
out_of_range = 1;
y = u;
